simulink model "PMDC_Controle_corrente"  (R2021a)
settings: Solver=ode4  StartTime=0.0  StopTime=0.020  FixedStep=0.00001  RelTol=1e-3
values from neighbouring files (symbols this model uses):
  B = 0    [P1_script.m]    (also in simulacao1.m)
  Ia_rated = 25    [P1_script.m]    (also in simulacao1.m)
  J = 0.001    [P1_script.m]    (also in simulacao1.m = 0.00252)
  Kac = 1/Kpc    (= 0.0936205547599)    [P1_script.m]
  Kic = Ra*2*pi*Wcc    (= 1633.62817987)    [P1_script.m]
  Kpc = La*2*pi*Wcc    (= 10.6814150222)    [P1_script.m]
  Kt = Te_rated/Ia_rated    (= 0.424752712124)    [P1_script.m]    (also in simulacao1.m)
  La = 1.7e-3    (= 0.0017)    [P1_script.m]    (also in simulacao1.m)
  Ra = 0.26    [P1_script.m]    (also in simulacao1.m)
settings Model: Creator=taylo  LastModifiedBy=taylo

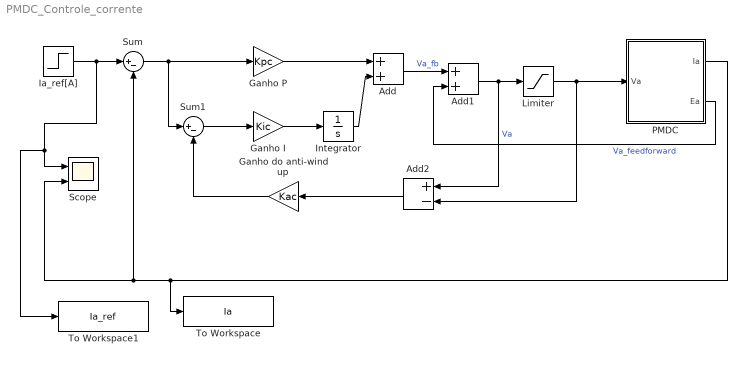
== system PMDC_Controle_corrente ==
  Add : Sum
  Add1 : Sum
  Add2 : Sum  Inputs=+-
  Ganho I : Gain  Gain=Kic
  Ganho P : Gain  Gain=Kpc
  Ganho do anti-wind up : Gain  Gain=Kac
  Ia_ref[A] : Step  Time=0.01  After=20  SampleTime=0
  Integrator : Integrator
  Limiter : Saturate  UpperLimit=Ia_rated  LowerLimit=-Ia_rated
  PMDC : Subsystem
  Scope : Scope  NumInputPorts=2
  Sum : Sum  Inputs=|+-
  Sum1 : Sum  Inputs=|+-
  To Workspace : ToWorkspace  VariableName=Ia  SaveFormat=Timeseries  SampleTime=-1
  To Workspace1 : ToWorkspace  VariableName=Ia_ref  SaveFormat=Timeseries  SampleTime=-1
  wires:
  Ia_ref[A]/1 -> To Workspace1/1, Scope/1, Sum/1
  Sum/1 -> Sum1/1, Ganho P/1
  Ganho P/1 -> Add/1
  Add/1 -> Add1/1  "Va_fb"
  Add1/1 -> Add2/1, Limiter/1  "Va"
  Limiter/1 -> Add2/2, PMDC/1(Va)
  PMDC/1(Ia) -> To Workspace/1, Scope/2, Sum/2
  Ganho I/1 -> Integrator/1
  Sum1/1 -> Ganho I/1
  Ganho do anti-wind up/1 -> Sum1/2
  Add2/1 -> Ganho do anti-wind up/1
  Integrator/1 -> Add/2
  PMDC/2(Ea) -> Add1/2  "Va_feedforward"

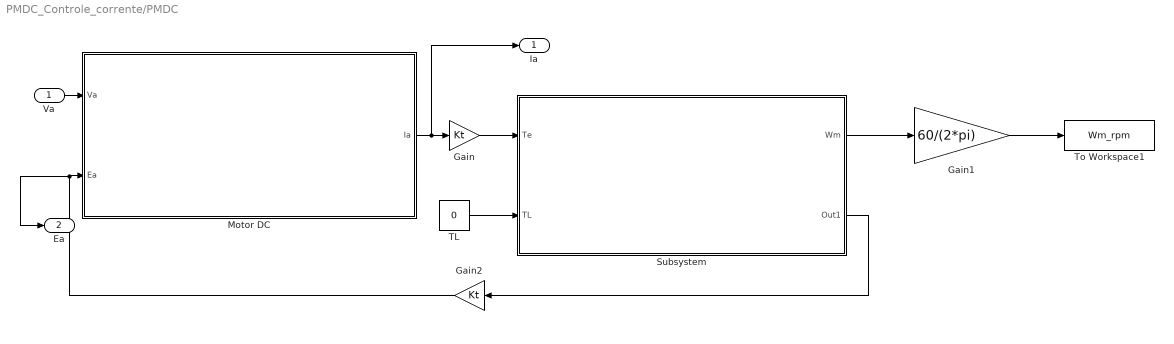
== system PMDC_Controle_corrente/PMDC ==
  Va : Inport
  Gain : Gain  Gain=Kt
  Gain1 : Gain  Gain=60/(2*pi)
  Gain2 : Gain  Gain=Kt
  Motor DC : Subsystem
  Subsystem : Subsystem
  TL : Constant  Value=0
  To Workspace1 : ToWorkspace  VariableName=Wm_rpm  SaveFormat=Timeseries  SampleTime=-1
  Ia : Outport
  Ea : Outport  Port=2
  wires:
  Motor DC/1(Ia) -> Ia/1, Gain/1
  Gain2/1 -> Ea/1, Motor DC/2(Ea)
  Gain/1 -> Subsystem/1(Te)
  Subsystem/1(Wm) -> Gain1/1
  Subsystem/2(Out1) -> Gain2/1
  TL/1 -> Subsystem/2(TL)
  Gain1/1 -> To Workspace1/1
  Va/1 -> Motor DC/1(Va)

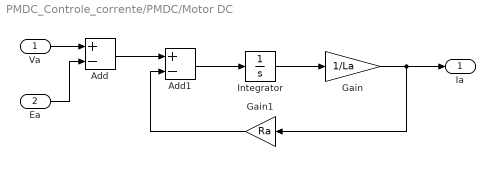
== system PMDC_Controle_corrente/PMDC/Motor DC ==
  Va : Inport
  Ea : Inport  Port=2
  Add : Sum  Inputs=+-
  Add1 : Sum  Inputs=+-
  Gain : Gain  Gain=1/La
  Gain1 : Gain  Gain=Ra
  Integrator : Integrator
  Ia : Outport
  wires:
  Add1/1 -> Integrator/1
  Gain1/1 -> Add1/2
  Add/1 -> Add1/1
  Va/1 -> Add/1
  Integrator/1 -> Gain/1
  Ea/1 -> Add/2
  Gain/1 -> Gain1/1, Ia/1

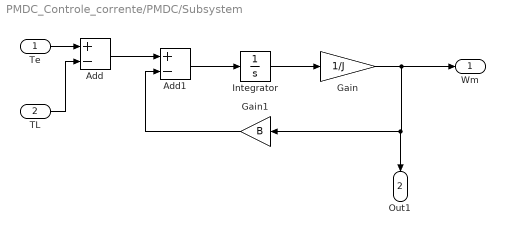
== system PMDC_Controle_corrente/PMDC/Subsystem ==
  Te : Inport
  TL : Inport  Port=2
  Add : Sum  Inputs=+-
  Add1 : Sum  Inputs=+-
  Gain : Gain  Gain=1/J
  Gain1 : Gain  Gain=B
  Integrator : Integrator
  Wm : Outport
  Out1 : Outport  Port=2
  wires:
  Te/1 -> Add/1
  Gain/1 -> Wm/1, Out1/1, Gain1/1
  Add/1 -> Add1/1
  TL/1 -> Add/2
  Add1/1 -> Integrator/1
  Gain1/1 -> Add1/2
  Integrator/1 -> Gain/1
